simulink model "trans_robostix"  (Simulink 7.1)
settings: Solver=FixedStepDiscrete  SolverMode=SingleTasking  StartTime=0.0  StopTime=inf  RelTol=1e-3
InitFcn:
  | trun = 1/50;
values from neighbouring files (symbols this model uses):
  count = count+1    (= 2)    [findVI.m]
libraries: xpcutilitieslib x13, xpclib x4
Description:
  | Serial Blocks Loopback Test Using Binary Encoding/Decoding
  | 
  | This model demonstrates the BINARY FIFO read block in a form that can be simulated without using any specific serial hardware.  The input to the FIFO write block is the concatenation of several pieces comprising two separate 'messages'.  The first message is the byte stream: [170, 1, N] and the second is [170 2 44 M] where N is an incrementing number and M is a decrementing number.  The initial '8' in the first constant is the number of elements that follow.  The '5' is an extraneous value that shows how the FIFO binary read will ignore extra information.
  | 
  | To run this test with real serial port hardware, replace the FIFO write block with the send/receive block with FIFO OUT that corresponds to your hardware from the xpclib rs232 section. Then feed the output signal back to the input with a wire to perform a loopback test.
settings Model: Creator=gweast  LastModifiedBy=Administrator  ExtModeArmWhenConnect=off  BufferReuse=off
settings DataIOCC: SaveOutput=off  SignalLogging=off  SaveTime=off
settings OptimizationCC: BlockReduction=off  OptimizeBlockIOStorage=off  BufferReuse=off  ExpressionFolding=off  FoldNonRolledExpr=off  LocalBlockOutputs=off
settings DebuggingCC: SaveWithParameterizedLinksMsg=none  SignalResolutionControl=TryResolveAllWithWarning  MultiTaskDSMMsg=warning  MultiTaskCondExecSysMsg=none  UnnecessaryDatatypeConvMsg=warning  StrictBusMsg=None
settings HardwareCC: ProdIntDivRoundTo=Zero  ProdEndianess=LittleEndian  ProdHWDeviceType=Generic->32-bit x86 compatible
settings RTWCC: SystemTargetFile=xpctarget.tlc  TemplateMakefile=xpc_default_tmf  Description=xPC Target  ProcessScript=xpctarget_make_rtw_hook  IncludeERTFirstTime=on
settings xpcTargetCC: TargetFcnLib=ansi_tfl_tmw.mat  TargetFunctionLibrary=ANSI_C  CompOptLevelCompliant=off  PortableWordSizes=off  xPCisDownloadable=off

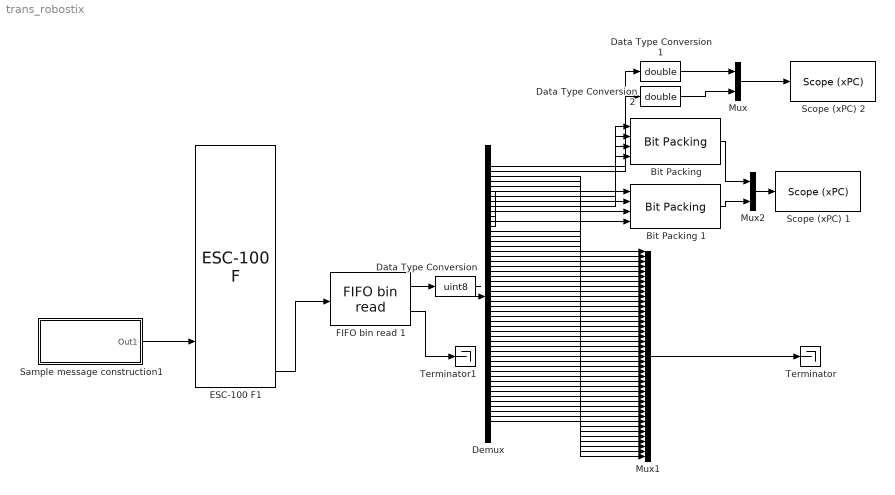
== system trans_robostix ==
  "Bit Packing " : xpcutilitieslib/Bit Packing   MaskBitPatterns={[0:7],[8:15],[16:23],[24:31]}  MaskPackDataType=single  MaskPackDataSize=[1]
  Bit Packing 1 : xpcutilitieslib/Bit Packing   MaskBitPatterns={[0:7],[8:15],[16:23],[24:31]}  MaskPackDataType=single  MaskPackDataSize=[1]
  Data Type Conversion : DataTypeConversion  OutDataTypeMode=uint8  OutDataType=sfix(16)  OutScaling=2^0  OutDataTypeStr=uint8
  Data Type Conversion1 : DataTypeConversion  OutDataTypeMode=double  OutDataType=sfix(16)  OutScaling=2^0  OutDataTypeStr=double
  Data Type Conversion2 : DataTypeConversion  OutDataTypeMode=double  OutDataType=sfix(16)  OutScaling=2^0  OutDataTypeStr=double
  Demux : Demux  Outputs=52
  ESC-100 F1 : xpclib/RS232/Quatech/ESC-100/ESC-100 F  SystemSampleTime=-1  group=FIFO Setup  port=7  irqnum=10  slot=-1  baud1=57600  parity1=None  ndata1=8  nstop1=1  fifomode1=64 deep  rlevel1=half full  automode1=off  xmtfifosize1=1024  xmtdatatype1=count+16 bit int  rcvfifosize1=1024  baud2=57600  parity2=None  ndata2=8  nstop2=1  fifomode2=64 deep  rlevel2=half full  automode2=off  xmtfifosize2=1024  xmtdatatype2=count+16 bit int  rcvfifosize2=1024  baud3=57600  parity3=None  ndata3=8  nstop3=1  fifomode3=64 deep  rlevel3=half full  automode3=off  xmtfifosize3=1024  xmtdatatype3=count+16 bit int  rcvfifosize3=1024  buad4=57600  parity4=None  ndata4=8  nstop4=1  fifomode4=64 deep  rlevel4=half full  automode4=off  xmtfifosize4=1024  xmtdatatype4=count+16 bit int  rcvfifosize4=1024  baud5=57600  parity5=None  ndata5=8  nstop5=1  fifomode5=64 deep  rlevel5=half full  automode5=off  xmtfifosize5=1024  xmtdatatype5=count+16 bit int  rcvfifosize5=1024  baud6=57600  parity6=None  ndata6=8  nstop6=1  fifomode6=64 deep  rlevel6=half full  automode6=off  xmtfifosize6=1024  xmtdatatype6=count+16 bit int  rcvfifosize6=1024  baud7=57600  parity7=None  ndata7=8  nstop7=1  fifomode7=64 deep  rlevel7=half full  automode7=off  xmtfifosize7=1024  xmtdatatype7=count+16 bit uint  rcvfifosize7=1024  baud8=57600  parity8=None  ndata8=8  nstop8=1  fifomode8=64 deep  rlevel8=half full  automode8=off  xmtfifosize8=1024  xmtdatatype8=count+16 bit uint  rcvfifosize8=1024
  FIFO bin read 1 : xpclib/RS232/FIFO bin read   header={char([147]), char([108])}  lengths=[48 4]  hold=Hold last output if no new data  enable=off  maxsize=51  outputtype=count+16 bit uint  sampletime=trun
  Mux : Mux  Inputs=2
  Mux1 : Mux  Inputs=43
  Mux2 : Mux  Inputs=2
  Sample message construction1 : Subsystem
  Scope (xPC) 1 : xpclib/Misc./Scope (xPC)   SystemSampleTime=-1  scopeno=2  scopetype=Target  autostart=on  viewmode=Graphical sliding  formatstr='%15.6f'  grid=on  ylimits=[0,0]  nosamples=512  noprepostsamples=0  interleave=1  triggermode=FreeRun  triggersignal=1  triggerlevel=0.0  triggerslope=Either  triggerscope=1  triggersample=0  filename=data.dat  mode=Lazy  writesize=512  autorestart=off
  Scope (xPC) 2 : xpclib/Misc./Scope (xPC)   SystemSampleTime=-1  scopeno=1  scopetype=Target  autostart=on  viewmode=Graphical sliding  formatstr='%15.6f'  grid=on  ylimits=[0,0]  nosamples=512  noprepostsamples=0  interleave=1  triggermode=FreeRun  triggersignal=1  triggerlevel=0.0  triggerslope=Either  triggerscope=1  triggersample=0  filename=data.dat  mode=Lazy  writesize=512  autorestart=off
  Terminator : Terminator
  Terminator1 : Terminator
  wires:
  FIFO bin read 1/1 -> Data Type Conversion/1
  Data Type Conversion/1 -> Demux/1
  Mux/1 -> Scope (xPC) 2/1
  Demux/1 -> Data Type Conversion1/1
  Demux/2 -> Data Type Conversion2/1
  Data Type Conversion1/1 -> Mux/1
  Data Type Conversion2/1 -> Mux/2
  Mux1/1 -> Terminator/1
  Demux/6 -> "Bit Packing "/1
  Demux/7 -> "Bit Packing "/2
  Demux/8 -> "Bit Packing "/3
  Demux/9 -> "Bit Packing "/4
  Demux/10 -> Bit Packing 1/1
  Demux/11 -> Bit Packing 1/2
  Demux/12 -> Bit Packing 1/3
  "Bit Packing "/1 -> Mux2/1
  Bit Packing 1/1 -> Mux2/2
  Mux2/1 -> Scope (xPC) 1/1
  Sample message construction1/1(Out1) -> ESC-100 F1/7
  ESC-100 F1/8 -> FIFO bin read 1/1
  FIFO bin read 1/2 -> Terminator1/1
  Demux/13 -> Bit Packing 1/4
  Demux/3 -> Mux1/1
  Demux/4 -> Mux1/2
  Demux/5 -> Mux1/3
  Demux/14 -> Mux1/4
  Demux/15 -> Mux1/5
  Demux/16 -> Mux1/6
  Demux/17 -> Mux1/7
  Demux/18 -> Mux1/8
  Demux/19 -> Mux1/9
  Demux/20 -> Mux1/10
  Demux/21 -> Mux1/11
  Demux/22 -> Mux1/12
  Demux/23 -> Mux1/13
  Demux/24 -> Mux1/14
  Demux/25 -> Mux1/15
  Demux/26 -> Mux1/16
  Demux/27 -> Mux1/17
  Demux/28 -> Mux1/18
  Demux/29 -> Mux1/19
  Demux/30 -> Mux1/20
  Demux/31 -> Mux1/21
  Demux/32 -> Mux1/22
  Demux/33 -> Mux1/23
  Demux/34 -> Mux1/24
  Demux/35 -> Mux1/25
  Demux/36 -> Mux1/26
  Demux/37 -> Mux1/27
  Demux/38 -> Mux1/28
  Demux/39 -> Mux1/29
  Demux/40 -> Mux1/30
  Demux/41 -> Mux1/31
  Demux/42 -> Mux1/32
  Demux/43 -> Mux1/33
  Demux/44 -> Mux1/34
  Demux/45 -> Mux1/35
  Demux/46 -> Mux1/36
  Demux/47 -> Mux1/37
  Demux/48 -> Mux1/38
  Demux/49 -> Mux1/39
  Demux/50 -> Mux1/40
  Demux/51 -> Mux1/41
  Demux/52 -> Mux1/42

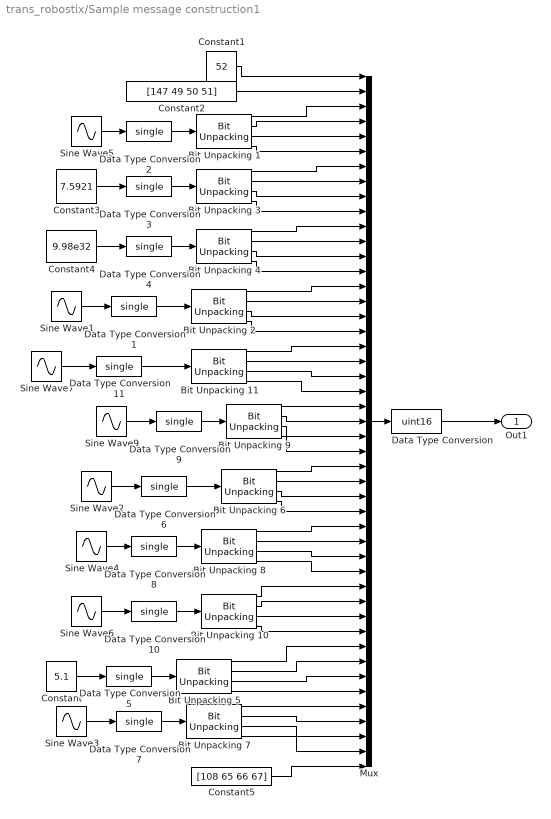
== system trans_robostix/Sample message construction1 ==
  Bit Unpacking {1..11} (11 alike) : xpcutilitieslib/Bit Unpacking   SignExtend=off  MaskBitPatterns={[0:7] , [8:15] , [16:23] , [24:31]}  MaskPackDataType=single  MaskPackDataSize=[1]  MaskUnpackDataTypes={'uint8','uint8','uint8','uint8'}  MaskUnpackDataSizes={[1],[1],[1],[1]}
  Constant : Constant  Value=5.1  OutDataTypeMode=single  OutDataType=sfix(16)  OutScaling=2^0  OutDataTypeStr=single
  Constant1 : Constant  Value=52  OutDataTypeMode=uint8  OutDataType=sfix(16)  OutScaling=2^0  OutDataTypeStr=uint8
  Constant2 : Constant  Value=[147 49 50 51]  OutDataTypeMode=uint8  OutDataType=sfix(16)  OutScaling=2^0  OutDataTypeStr=uint8
  Constant3 : Constant  Value=7.5921  OutDataTypeMode=single  OutDataType=sfix(16)  OutScaling=2^0  OutDataTypeStr=single
  Constant4 : Constant  Value=9.98e32  OutDataTypeMode=single  OutDataType=sfix(16)  OutScaling=2^0  OutDataTypeStr=single
  Constant5 : Constant  Value=[108 65 66 67]  OutDataTypeMode=uint8  OutDataType=sfix(16)  OutScaling=2^0  OutDataTypeStr=uint8
  Data Type Conversion : DataTypeConversion  OutDataTypeMode=uint16  OutDataType=sfix(16)  OutScaling=2^0  OutDataTypeStr=uint16  ConvertRealWorld=Stored Integer (SI)
  Data Type Conversion{1..11} (11 alike) : DataTypeConversion  OutDataTypeMode=single  OutDataType=sfix(16)  OutScaling=2^0  OutDataTypeStr=single
  Mux : Mux  Inputs=47
  Sine Wave1 : Sin  Frequency=4  Phase=pi/4  SampleTime=trun
  Sine Wave2 : Sin  Frequency=2  Phase=pi/4  SampleTime=trun
  Sine Wave3 : Sin  Frequency=16  Phase=pi/4  SampleTime=trun
  Sine Wave4 : Sin  Phase=pi/4  SampleTime=trun
  Sine Wave5 : Sin  Frequency=4  Phase=pi/4  SampleTime=trun
  Sine Wave6 : Sin  Frequency=2  SampleTime=trun
  Sine Wave7 : Sin  Frequency=1.2  SampleTime=trun
  Sine Wave9 : Sin  Frequency=16  Phase=pi/4  SampleTime=trun
  Out1 : Outport  OutDataType=sfix(16)  OutScaling=2^0
  wires:
  Mux/1 -> Data Type Conversion/1
  Sine Wave5/1 -> Data Type Conversion2/1
  Constant3/1 -> Data Type Conversion3/1
  Constant4/1 -> Data Type Conversion4/1
  Data Type Conversion2/1 -> Bit Unpacking 1/1
  Data Type Conversion3/1 -> Bit Unpacking 3/1
  Data Type Conversion4/1 -> Bit Unpacking 4/1
  Data Type Conversion/1 -> Out1/1
  Constant1/1 -> Mux/1
  Constant2/1 -> Mux/2
  Bit Unpacking 1/1 -> Mux/3
  Bit Unpacking 1/2 -> Mux/4
  Bit Unpacking 1/3 -> Mux/5
  Bit Unpacking 1/4 -> Mux/6
  Bit Unpacking 3/1 -> Mux/7
  Bit Unpacking 3/2 -> Mux/8
  Bit Unpacking 3/3 -> Mux/9
  Bit Unpacking 3/4 -> Mux/10
  Bit Unpacking 4/1 -> Mux/11
  Bit Unpacking 4/2 -> Mux/12
  Bit Unpacking 4/3 -> Mux/13
  Bit Unpacking 4/4 -> Mux/14
  Sine Wave1/1 -> Data Type Conversion1/1
  Data Type Conversion1/1 -> Bit Unpacking 2/1
  Bit Unpacking 2/1 -> Mux/15
  Bit Unpacking 2/2 -> Mux/16
  Bit Unpacking 2/3 -> Mux/17
  Bit Unpacking 2/4 -> Mux/18
  Sine Wave2/1 -> Data Type Conversion6/1
  Data Type Conversion6/1 -> Bit Unpacking 6/1
  Sine Wave9/1 -> Data Type Conversion9/1
  Data Type Conversion9/1 -> Bit Unpacking 9/1
  Bit Unpacking 9/1 -> Mux/23
  Bit Unpacking 9/2 -> Mux/24
  Bit Unpacking 9/3 -> Mux/25
  Bit Unpacking 9/4 -> Mux/26
  Bit Unpacking 6/1 -> Mux/27
  Bit Unpacking 6/2 -> Mux/28
  Bit Unpacking 6/3 -> Mux/29
  Bit Unpacking 6/4 -> Mux/30
  Sine Wave3/1 -> Data Type Conversion7/1
  Data Type Conversion7/1 -> Bit Unpacking 7/1
  Sine Wave4/1 -> Data Type Conversion8/1
  Sine Wave6/1 -> Data Type Conversion10/1
  Data Type Conversion8/1 -> Bit Unpacking 8/1
  Data Type Conversion10/1 -> Bit Unpacking 10/1
  Bit Unpacking 8/1 -> Mux/31
  Bit Unpacking 8/2 -> Mux/32
  Bit Unpacking 8/3 -> Mux/33
  Bit Unpacking 8/4 -> Mux/34
  Bit Unpacking 10/1 -> Mux/35
  Bit Unpacking 10/2 -> Mux/36
  Bit Unpacking 10/3 -> Mux/37
  Bit Unpacking 10/4 -> Mux/38
  Bit Unpacking 7/1 -> Mux/43
  Bit Unpacking 7/2 -> Mux/44
  Bit Unpacking 7/3 -> Mux/45
  Bit Unpacking 7/4 -> Mux/46
  Constant5/1 -> Mux/47
  Sine Wave7/1 -> Data Type Conversion11/1
  Data Type Conversion11/1 -> Bit Unpacking 11/1
  Constant/1 -> Data Type Conversion5/1
  Data Type Conversion5/1 -> Bit Unpacking 5/1
  Bit Unpacking 11/1 -> Mux/19
  Bit Unpacking 11/2 -> Mux/20
  Bit Unpacking 11/3 -> Mux/21
  Bit Unpacking 11/4 -> Mux/22
  Bit Unpacking 5/1 -> Mux/39
  Bit Unpacking 5/2 -> Mux/40
  Bit Unpacking 5/3 -> Mux/41
  Bit Unpacking 5/4 -> Mux/42
